simulink model "LOWPASSFILTER"  (R2016a)
settings: Solver=FixedStepAuto  StartTime=1  StopTime=601  RelTol=1e-3
libraries: simulink x4, dspsigops x1
settings Model: Creator=Bilal  LastModifiedBy=Bilal

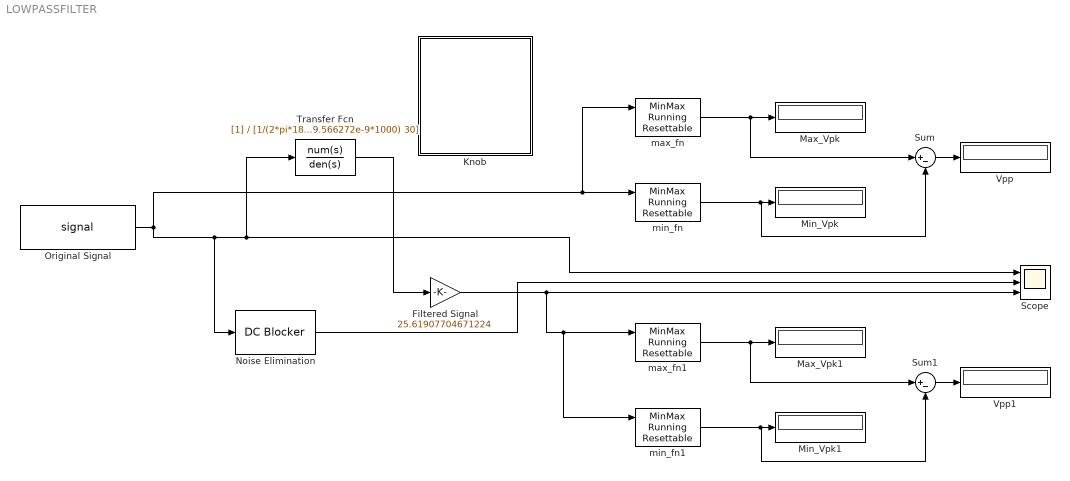
== system LOWPASSFILTER ==
  Filtered Signal : Gain  Gain=25.61907704671224
  Knob : Subsystem  DialogController=hmiCreateDDGDialog  IsWebBlock=on  mask(MWDashboardBlock){webBlockId=ad41e934-75c8-4f3f-acde-8a855f4ad45f, webBlockType=continuousknob, ShowInLibBrowser=on, ShowInitialText=on, HMISrcModelName=LOWPASSFILTER}
      mask prompts: webBlockId "WebBlock Id"; webBlockType "WebBlock Type"; HMISrcModelName "Source Model"
      mask Help: helpview([docroot '/mapfiles/simulink.map'], 'hmi_knob')
      mask Display:
      | if strcmp(get_param(bdroot(gcb),'BlockDiagramType'), 'library')
      |     image([(matlabroot) '/toolbox/simulink/hmi/icons/ContinuousKnob.png']);
      | end
  Max_Vpk : Display
  Max_Vpk1 : Display
  Min_Vpk : Display
  Min_Vpk1 : Display
  Noise Elimination : dspsigops/DC Blocker  Algorithm=FIR  NormalizedBandwidth=0.001  Length=8  Order=6  SimulateUsing=Code generation
  Original Signal : FromWorkspace  VariableName=signal  SampleTime=1
  Scope : Scope  NumInputPorts=3
  Sum : Sum  Inputs=|+-
  Sum1 : Sum  Inputs=|+-
  Transfer Fcn : TransferFcn  Denominator=[1/(2*pi*189.566272e-9*1000) 30]
  Vpp : Display
  Vpp1 : Display
  max_fn : simulink/Math Operations/MinMax Running Resettable  Function=max  vinit=0.0
  max_fn1 : simulink/Math Operations/MinMax Running Resettable  Function=max  vinit=0.0
  min_fn : simulink/Math Operations/MinMax Running Resettable  Function=min  vinit=0.0
  min_fn1 : simulink/Math Operations/MinMax Running Resettable  Function=min  vinit=0.0
  wires:
  Noise Elimination/1 -> Scope/2
  min_fn/1 -> Sum/2, Min_Vpk/1
  Original Signal/1 -> Noise Elimination/1, Scope/1, Transfer Fcn/1, max_fn/1, min_fn/1
  max_fn/1 -> Sum/1, Max_Vpk/1
  Sum/1 -> Vpp/1
  Transfer Fcn/1 -> Filtered Signal/1
  min_fn1/1 -> Sum1/2, Min_Vpk1/1
  Filtered Signal/1 -> min_fn1/1, max_fn1/1, Scope/3
  max_fn1/1 -> Sum1/1, Max_Vpk1/1
  Sum1/1 -> Vpp1/1

== system LOWPASSFILTER/Knob ==
